simulink model "Consensus_HP_test_avg_noise"  (R2022a)
settings: Solver=VariableStepAuto  StartTime=0.0  StopTime=50  RelTol=1e-3
InitFcn:
  | dt=0.0001;
  | 
  | 
  | L=[1 -1;-1 1];
  | L = [ 2 -1  0 -1; -1  2 -1  0; 0 -1  2 -1; -1  0 -1  2];
  | [n,~]=size(L);
  | beta=100;
  | L=beta*L;
  | L=kron(L,eye(m));
  | n=n*2;
libraries: cstblocks x1
settings Model: Creator=Lirui  LastModifiedBy=Lirui

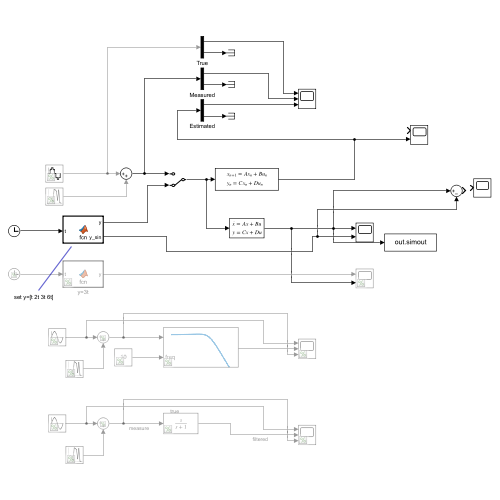
[thumbnail: Simulink's stored preview of the top-level diagram]
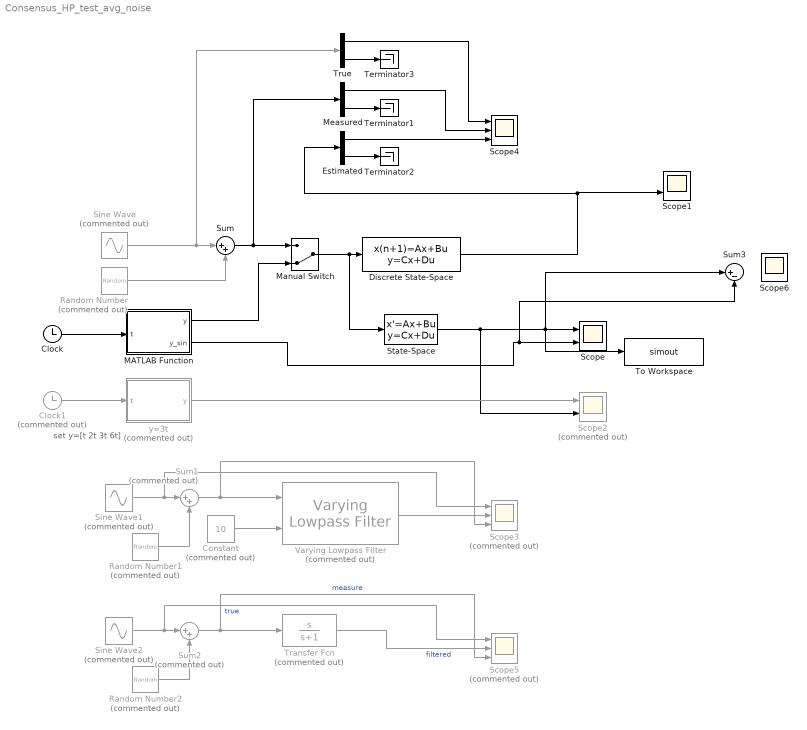
== system Consensus_HP_test_avg_noise ==
  note: set y=[t 2t 3t 6t]
  Clock : Clock
  Clock1 : Clock  Commented=on
  Constant : Constant  Commented=on  Value=10
  Discrete State-Space : DiscreteStateSpace  A=eye(n)-dt*L  B=-dt*L  C=eye(n)  D=eye(n)  InitialCondition=zeros(n,1)  SampleTime=dt
  Estimated : Demux  Outputs=[1 n-1]
  MATLAB Function : MATLAB Function  TreatAsAtomicUnit=on
  Manual Switch : ManualSwitch  CurrentSetting=0
  Measured : Demux  Outputs=[1 n-1]
  Random Number : RandomNumber  Commented=on  Variance=0.0001*ones(n,1)  Seed=randi([1, 100], n, 1);  SampleTime=dt
  Random Number1 : RandomNumber  Commented=on
  Random Number2 : RandomNumber  Commented=on
  Scope : Scope  NumInputPorts=2
  Scope1 : Scope  NumInputPorts=2
  Scope2 : Scope  Commented=on  NumInputPorts=2
  Scope3 : Scope  Commented=on  NumInputPorts=3
  Scope4 : Scope  NumInputPorts=3
  Scope5 : Scope  Commented=on  NumInputPorts=3
  Scope6 : Scope
  Sine Wave : Sin  Commented=on  Amplitude=1*ones(n,1)  Bias=[1 2 3 6]'  Frequency=1*ones(n,1)  SampleTime=dt
  Sine Wave1 : Sin  Commented=on  SampleTime=0
  Sine Wave2 : Sin  Commented=on  Frequency=5  SampleTime=0
  State-Space : StateSpace  A=-L  B=-L  C=eye(n)  D=eye(n)  InitialCondition=zeros(n,1)
  Sum : Sum  Inputs=|++
  Sum1 : Sum  Commented=on  Inputs=|++
  Sum2 : Sum  Commented=on  Inputs=|++
  Sum3 : Sum  Inputs=|+-
  Terminator1 : Terminator
  Terminator2 : Terminator
  Terminator3 : Terminator
  To Workspace : ToWorkspace  VariableName=simout  SaveFormat=Timeseries  SampleTime=-1
  Transfer Fcn : TransferFcn  Commented=on  Numerator=[1 0]  Denominator=[1 1]
  True : Demux  Outputs=[1 n-1]
  Varying Lowpass Filter : cstblocks/Linear Parameter Varying/Varying Lowpass Filter  Commented=on  N=4
  y=3t : MATLAB Function  Commented=on  TreatAsAtomicUnit=on
  wires:
  Clock/1 -> MATLAB Function/1(t)
  Discrete State-Space/1 -> Estimated/1, Scope1/2
  Random Number/1 -> Sum/2
  Sine Wave/1 -> True/1, Sum/1
  Sum/1 -> Manual Switch/1, Measured/1
  Clock1/1 -> y=3t/1(t)
  State-Space/1 -> Scope2/2, Sum3/1, Scope/1, To Workspace/1
  y=3t/1(y) -> Scope2/1
  Measured/2 -> Terminator1/1
  Measured/1 -> Scope4/2
  Estimated/1 -> Scope4/3
  Estimated/2 -> Terminator2/1
  True/2 -> Terminator3/1
  True/1 -> Scope4/1
  MATLAB Function/1(y) -> Manual Switch/2
  Manual Switch/1 -> State-Space/1, Discrete State-Space/1
  Constant/1 -> Varying Lowpass Filter/2
  Varying Lowpass Filter/1 -> Scope3/2
  Sine Wave1/1 -> Scope3/1, Sum1/1
  Sum1/1 -> Scope3/3, Varying Lowpass Filter/1
  Random Number1/1 -> Sum1/2
  Transfer Fcn/1 -> Scope5/2  "filtered"
  Random Number2/1 -> Sum2/2
  Sum2/1 -> Transfer Fcn/1, Scope5/3  "measure"
  Sine Wave2/1 -> Scope5/1, Sum2/1  "true"
  MATLAB Function/2(y_sin) -> Sum3/2, Scope/2

== matlab function Consensus_HP_test_avg_noise/MATLAB Function ==
  data: t input; y output; y_sin output
function [y,y_sin] = fcn(t)
w=10;
%y=[sin(w*t)+1,sin(w*t)+2,sin(w*t)+3,sin(w*t)+6]';

%y=[sin(w*t)+1,sin(w*t)+2,sin(w*t)+3,sin(w*t)+6]';
%y=[40*sin(w*t),0,0,0]';
y=[1*sin(w*t),0,      1*sin(w*t),0,     0,5*sin(w*t),    0,5*sin(w*t)]';
y_sin=1*sin(w*t);

%y=[exp(-t)+1,exp(-t)+2,exp(-t)+3,exp(-t)+6]';

%y=[10 20 30 60]';

%y=[t 2*t 3*t 6*t]';
%y=[t+1 2*t+2 3*t+3 6*t+6]';

%y=[t+1 t+2 t+3 t+6]'; % this one is tested in the original paper

== matlab function Consensus_HP_test_avg_noise/y=3t ==
  data: t input; y output
function y = fcn(t)


y=3*t;
%y=3*t+3;
